simulink model "csu_imk_imu_kinematics_hrn_a"  (R2014b)
settings: Solver=FixedStepDiscrete  StartTime=0.0  StopTime=2  FixedStep=1  RelTol=1e-3
libraries: csu_imk_imu_kinematics_lib_a x1, util_quat_lib x1
settings Model: BufferReuse=off  Creator=hcannon  LastModifiedBy=mstewart
settings DataIOCC: SignalLoggingSaveFormat=ModelDataLogs
settings OptimizationCC: OptimizeBlockIOStorage=off  BufferReuse=off  GlobalBufferReuse=off  ExpressionFolding=off  ExpressionDepthLimit=2147483647  LocalBlockOutputs=off  InitFltsAndDblsToZero=on
settings DebuggingCC: UnderspecifiedInitializationDetection=Classic  MergeDetectMultiDrivingBlocksExec=none  FcnCallInpInsideContextMsg=UseLocalSettings  StateNameClashWarn=warning  StrictBusMsg=Warning
settings GRTTargetCC: CombineOutputUpdateFcns=off  GRTInterface=on

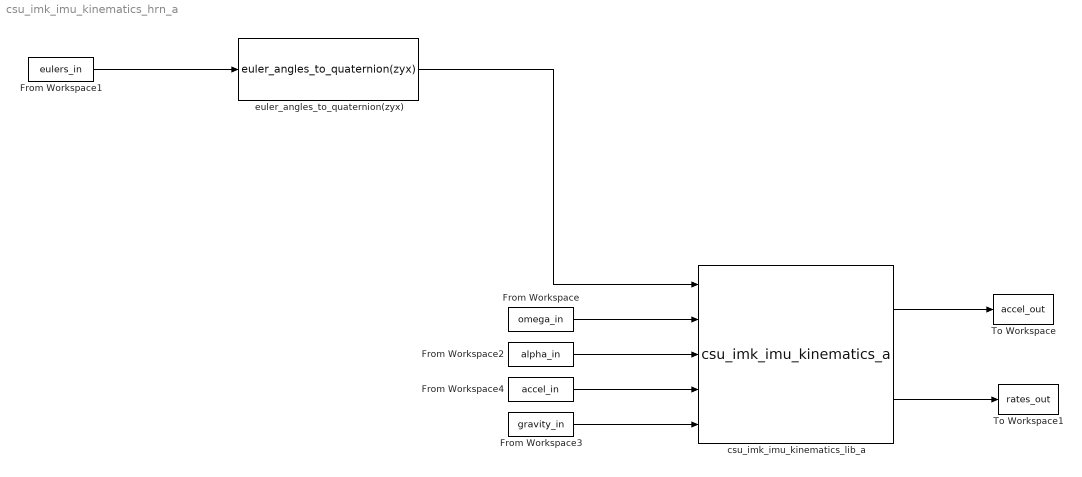
== system csu_imk_imu_kinematics_hrn_a ==
  From Workspace : FromWorkspace  VariableName=omega_in  SampleTime=0
  From Workspace1 : FromWorkspace  VariableName=eulers_in  SampleTime=0
  From Workspace2 : FromWorkspace  VariableName=alpha_in  SampleTime=0
  From Workspace3 : FromWorkspace  VariableName=gravity_in  SampleTime=0
  From Workspace4 : FromWorkspace  VariableName=accel_in  SampleTime=0
  To Workspace : ToWorkspace  VariableName=accel_out  SampleTime=-1
  To Workspace1 : ToWorkspace  VariableName=rates_out  SampleTime=-1
  csu_imk_imu_kinematics_lib_a : csu_imk_imu_kinematics_lib_a/csu_imk_imu_kinematics_a
  euler_angles_to_quaternion(zyx) : util_quat_lib/euler_angles_to_quaternion(zyx)  SystemSampleTime=-1
  wires:
  csu_imk_imu_kinematics_lib_a/1 -> To Workspace/1
  csu_imk_imu_kinematics_lib_a/2 -> To Workspace1/1
  From Workspace2/1 -> csu_imk_imu_kinematics_lib_a/3
  From Workspace1/1 -> euler_angles_to_quaternion(zyx)/1
  From Workspace3/1 -> csu_imk_imu_kinematics_lib_a/5
  From Workspace/1 -> csu_imk_imu_kinematics_lib_a/2
  euler_angles_to_quaternion(zyx)/1 -> csu_imk_imu_kinematics_lib_a/1
  From Workspace4/1 -> csu_imk_imu_kinematics_lib_a/4
